simulink model "F18_sim_debug"  (R2025b)
settings: Solver=VariableStepAuto  StartTime=0.0  StopTime=10.0  RelTol=1e-3
undefined symbols (not defined in the file): F18
settings Model: Creator=deepa  LastModifiedBy=deepa

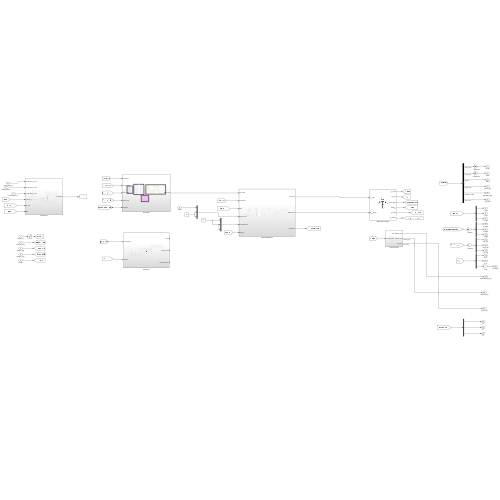
[thumbnail: Simulink's stored preview of the top-level diagram]
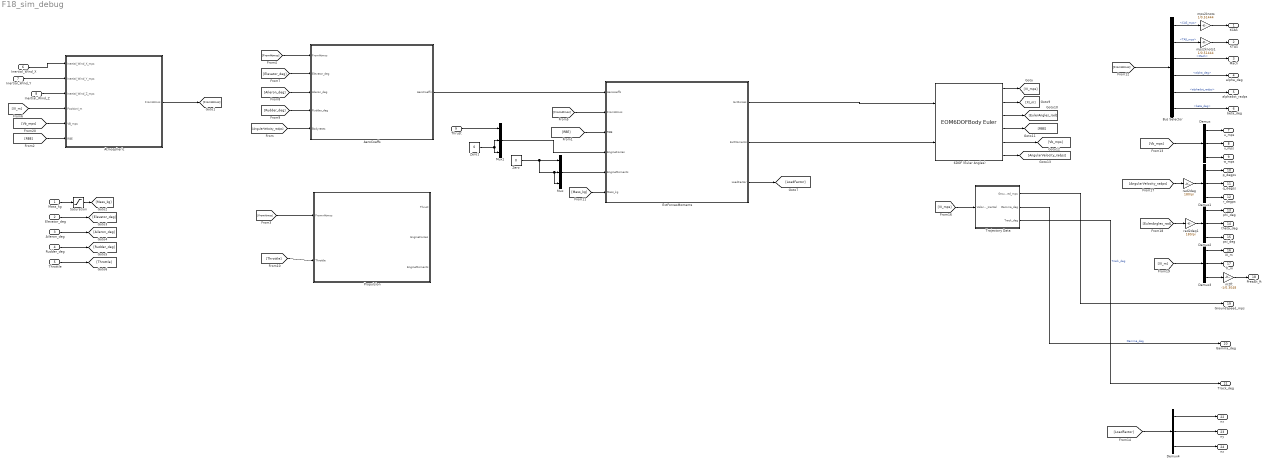
== system F18_sim_debug ==
  Mass_kg : Inport
  Elevator_deg : Inport  Port=2
  Aileron_deg : Inport  Port=3
  Rudder_deg : Inport  Port=4
  Throttle : Inport  Port=5
  Inertial_Wind_X : Inport  Port=6
  Inertial_Wind_Y : Inport  Port=7
  Inertial_Wind_Z : Inport  Port=8
  Thrust : Inport  Port=9
  6DOF (Euler Angles) : EOM6DOFBodyEuler  mass_0=15118.35  inertia=F18.Inertia  Vm_statename={'u_mps','v_mps','z_mps'}  xme_statename={'XI_m','YI_m','ZI_m'}  pm_statename={'p_radps','q_rapds','r_radps'}  eul_statename={'phi_rad','theta_rad','psi_rad'}
  AeroCoeffs : Subsystem
  Atmospheric : Subsystem
  Bus Selector : BusSelector  OutputSignals=CAS_mps,TAS_mps,Mach,alpha_deg,alphadot_radps,beta_deg
  Demux{,1..4} (5 alike) : Demux  Outputs=3
  ExtForcesMoments : Subsystem
  Mux : Mux  Inputs=3
  Mux1 : Mux  Inputs=3
  Propulsion : Subsystem
  Saturation : Saturate  UpperLimit=inf  LowerLimit=0.1
  Trajectory Data : Subsystem
  Zero : Constant  Value=0  OutDataTypeStr=Inherit: Inherit via back propagation
  Zero1 : Constant  Value=0  OutDataTypeStr=Inherit: Inherit via back propagation
  m2ft : Gain  Gain=-1/0.3048
  mps2knots : Gain  Gain=1/0.51444
  mps2knots1 : Gain  Gain=1/0.51444
  rad2deg : Gain  Gain=180/pi
  rad2deg1 : Gain  Gain=180/pi
  KCAS : Outport
  KTAS : Outport  Port=2
  Mach : Outport  Port=3
  alpha_deg : Outport  Port=4
  alphadot_radps : Outport  Port=5
  beta_deg : Outport  Port=6
  u_mps : Outport  Port=7
  v_mps : Outport  Port=8
  w_mps : Outport  Port=9
  p_degps : Outport  Port=10
  q_degps : Outport  Port=11
  r_degps : Outport  Port=12
  phi_deg : Outport  Port=13
  theta_deg : Outport  Port=14
  psi_deg : Outport  Port=15
  XI_m : Outport  Port=16
  YI_m : Outport  Port=17
  PresAlt_ft : Outport  Port=18
  GroundSpeed_mps : Outport  Port=19
  Gamma_deg : Outport  Port=20
  Track_deg : Outport  Port=21
  nx : Outport  Port=22
  ny : Outport  Port=23
  nz : Outport  Port=24
  wires:
  Bus Selector/3 -> Mach/1  "<Mach>"
  Saturation/1 -> [Mass_kg]
  Throttle/1 -> [Throttle]
  Aileron_deg/1 -> [Aileron_deg]
  [Elevator_deg] -> AeroCoeffs/2(Elevator_deg)
  Mass_kg/1 -> Saturation/1
  Inertial_Wind_X/1 -> Atmospheric/1(Inertial_Wind_X_mps)
  Trajectory Data/1(GroundSpeed_mps) -> GroundSpeed_mps/1
  [XI_m] -> Demux3/1
  AeroCoeffs/1(AeroCoeffs) -> ExtForcesMoments/1(Aerocoeffs)
  ExtForcesMoments/2(ExtMoments) -> 6DOF (Euler Angles)/2
  Demux2/3 -> psi_deg/1
  [Aileron_deg] -> AeroCoeffs/3(Aileron_deg)
  Bus Selector/1 -> mps2knots/1  "<CAS_mps>"
  Atmospheric/1(FromAtmos) -> [FromAtmos]
  Demux4/1 -> nx/1
  Demux1/3 -> r_degps/1
  rad2deg1/1 -> Demux2/1
  [LoadFactor] -> Demux4/1
  Rudder_deg/1 -> [Rudder_deg]
  Elevator_deg/1 -> [Elevator_deg]
  Demux3/1 -> XI_m/1
  Bus Selector/6 -> beta_deg/1  "<beta_deg>"
  Demux4/2 -> ny/1
  Demux3/2 -> YI_m/1
  Demux2/1 -> phi_deg/1
  Inertial_Wind_Y/1 -> Atmospheric/2(Inertial_Wind_Y_mps)
  Demux4/3 -> nz/1
  Bus Selector/4 -> alpha_deg/1  "<alpha_deg>"
  Demux3/3 -> m2ft/1
  Demux1/2 -> q_degps/1
  mps2knots/1 -> KCAS/1
  Inertial_Wind_Z/1 -> Atmospheric/3(Inertial_Wind_Z_mps)
  rad2deg/1 -> Demux1/1
  [Vb_mps] -> Demux/1
  [FromAtmos] -> Propulsion/1(FromnAtmos)
  Bus Selector/5 -> alphadot_radps/1  "<alphadot_radps>"
  [AngularVelocity_radps] -> rad2deg/1
  [EulerAngles_rad] -> rad2deg1/1
  [Mass_kg] -> ExtForcesMoments/6(Mass_kg)
  [Rudder_deg] -> AeroCoeffs/4(Rudder_deg)
  Demux/2 -> v_mps/1
  [RBE] -> ExtForcesMoments/3(RBE)
  [Throttle] -> Propulsion/2(Throttle)
  [FromAtmos] -> ExtForcesMoments/2(FromAtmos)
  [AngularVelocity_radps] -> AeroCoeffs/5(Bodyrates)
  Demux/3 -> w_mps/1
  ExtForcesMoments/3(LoadFactor) -> [LoadFactor]
  [FromAtmos] -> AeroCoeffs/1(FromAtmos)
  Demux1/1 -> p_degps/1
  Bus Selector/2 -> mps2knots1/1  "<TAS_mps>"
  m2ft/1 -> PresAlt_ft/1
  Demux/1 -> u_mps/1
  [FromAtmos] -> Bus Selector/1
  ExtForcesMoments/1(ExtForces) -> 6DOF (Euler Angles)/1
  Demux2/2 -> theta_deg/1
  mps2knots1/1 -> KTAS/1
  6DOF (Euler Angles)/1 -> [VI_mps]
  6DOF (Euler Angles)/2 -> [XI_m]
  6DOF (Euler Angles)/3 -> [EulerAngles_rad]
  6DOF (Euler Angles)/4 -> [RBE]
  6DOF (Euler Angles)/5 -> [Vb_mps]
  6DOF (Euler Angles)/6 -> [AngularVelocity_radps]
  [RBE] -> Atmospheric/6(RBE)
  [XI_m] -> Atmospheric/4(PositionI_m)
  [VI_mps] -> Trajectory Data/1(Velocity_Inertial)
  Trajectory Data/2(Gamma_deg) -> Gamma_deg/1  "Gamma_deg"
  Trajectory Data/3(Track_deg) -> Track_deg/1  "Track_deg"
  [Vb_mps] -> Atmospheric/5(VB_mps)
  Zero/1 -> Mux/3, Mux/2, Mux/1
  Mux/1 -> ExtForcesMoments/5(EngineMoments)
  Thrust/1 -> Mux1/1
  Zero1/1 -> Mux1/2, Mux1/3
  Mux1/1 -> ExtForcesMoments/4(EngineForces)

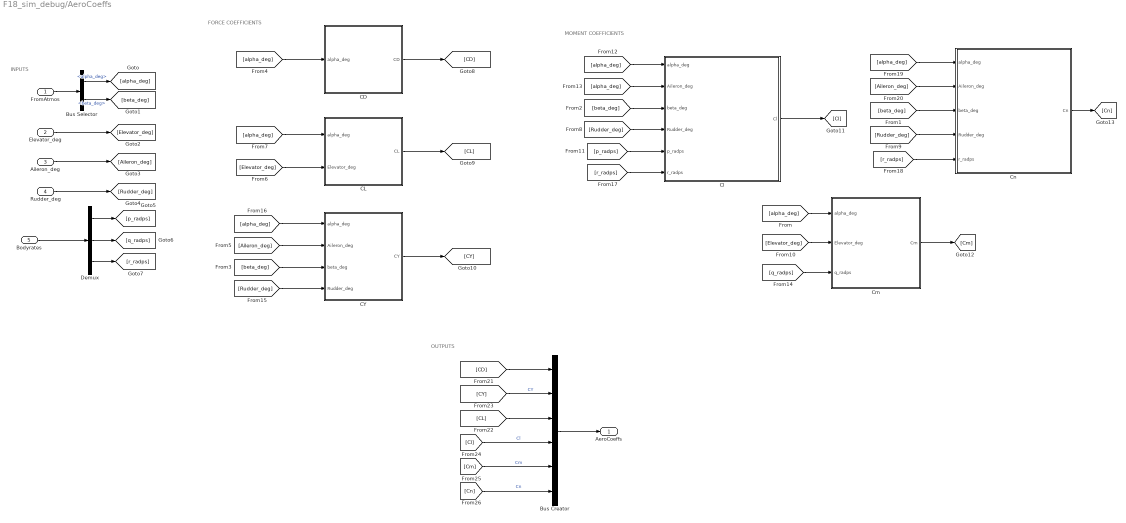
== system F18_sim_debug/AeroCoeffs ==
  note: OUTPUTS
  note: MOMENT COEFFICIENTS
  note: FORCE COEFFICIENTS
  note: INPUTS
  FromAtmos : Inport
  Elevator_deg : Inport  Port=2
  Aileron_deg : Inport  Port=3
  Rudder_deg : Inport  Port=4
  Bodyrates : Inport  Port=5
  Bus Creator : BusCreator  Inputs=6
  Bus Selector : BusSelector  OutputSignals=alpha_deg,beta_deg
  CD : Subsystem
  CL : Subsystem
  CY : Subsystem
  Cl : Subsystem
  Cm : Subsystem
  Cn : Subsystem
  Demux : Demux  Outputs=3
  AeroCoeffs : Outport
  wires:
  FromAtmos/1 -> Bus Selector/1
  [alpha_deg] -> Cm/1(alpha_deg)
  [beta_deg] -> Cn/3(beta_deg)
  [beta_deg] -> Cl/3(beta_deg)
  [beta_deg] -> CY/3(beta_deg)
  [alpha_deg] -> CD/1(alpha_deg)
  Elevator_deg/1 -> [Elevator_deg]
  Aileron_deg/1 -> [Aileron_deg]
  Rudder_deg/1 -> [Rudder_deg]
  [Aileron_deg] -> CY/2(Aileron_deg)
  [Elevator_deg] -> CL/2(Elevator_deg)
  [alpha_deg] -> CL/1(alpha_deg)
  [Rudder_deg] -> Cl/4(Rudder_deg)
  [Rudder_deg] -> Cn/4(Rudder_deg)
  [Elevator_deg] -> Cm/2(Elevator_deg)
  Bodyrates/1 -> Demux/1
  Demux/1 -> [p_radps]
  Demux/2 -> [q_radps]
  Demux/3 -> [r_radps]
  [p_radps] -> Cl/5(p_radps)
  [alpha_deg] -> Cl/1(alpha_deg)
  [alpha_deg] -> Cl/2(Aileron_deg)
  [q_radps] -> Cm/3(q_radps)
  [Rudder_deg] -> CY/4(Rudder_deg)
  [alpha_deg] -> CY/1(alpha_deg)
  [r_radps] -> Cl/6(r_radps)
  [r_radps] -> Cn/5(r_radps)
  [alpha_deg] -> Cn/1(alpha_deg)
  [Aileron_deg] -> Cn/2(Aileron_deg)
  CD/1(CD) -> [CD]
  CL/1(CL) -> [CL]
  CY/1(CY) -> [CY]
  Cl/1(Cl) -> [Cl]
  Cm/1(Cm) -> [Cm]
  Cn/1(Cn) -> [Cn]
  [CD] -> Bus Creator/1
  [CY] -> Bus Creator/2  "CY"
  [CL] -> Bus Creator/3
  [Cn] -> Bus Creator/6  "Cn"
  [Cm] -> Bus Creator/5  "Cm"
  [Cl] -> Bus Creator/4  "Cl"
  Bus Creator/1 -> AeroCoeffs/1
  Bus Selector/1 -> [alpha_deg]  "<alpha_deg>"
  Bus Selector/2 -> [beta_deg]  "<beta_deg>"

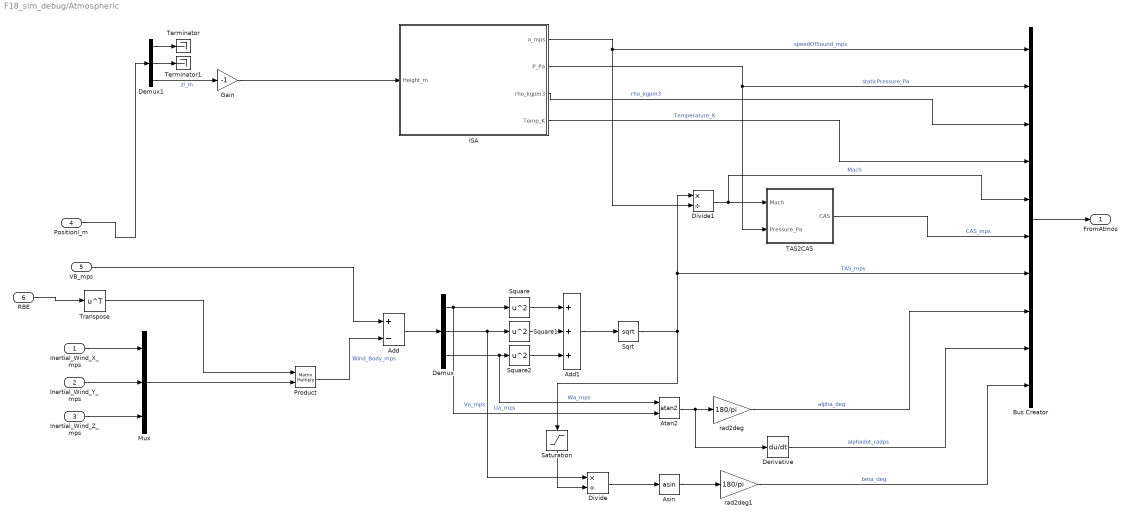
== system F18_sim_debug/Atmospheric ==
  Inertial_Wind_X_mps : Inport
  Inertial_Wind_Y_mps : Inport  Port=2
  Inertial_Wind_Z_mps : Inport  Port=3
  PositionI_m : Inport  Port=4
  VB_mps : Inport  Port=5
  RBE : Inport  Port=6
  Add : Sum  Inputs=+-
  Add1 : Sum  Inputs=+++
  Asin : Trigonometry  Operator=asin
  Atan2 : Trigonometry  Operator=atan2
  Bus Creator : BusCreator  Inputs=10
  Demux : Demux  Outputs=3
  Demux1 : Demux  Outputs=3
  Derivative : Derivative
  Divide : Product  Inputs=*/
  Divide1 : Product  Inputs=*/
  Gain : Gain  Gain=-1
  ISA : Subsystem
  Mux : Mux  Inputs=3
  Product : Product  Multiplication=Matrix(*)
  Saturation : Saturate  UpperLimit=inf  LowerLimit=0.1
  Sqrt : Sqrt
  Square : Math  Operator=square
  Square1 : Math  Operator=square
  Square2 : Math  Operator=square
  TAS2CAS : Subsystem
  Terminator : Terminator
  Terminator1 : Terminator
  Transpose : Math  Operator=transpose
  rad2deg : Gain  Gain=180/pi
  rad2deg1 : Gain  Gain=180/pi
  FromAtmos : Outport
  wires:
  Gain/1 -> ISA/1(Height_m)
  VB_mps/1 -> Add/1
  PositionI_m/1 -> Demux1/1
  Demux1/1 -> Terminator/1
  Demux1/2 -> Terminator1/1
  Demux1/3 -> Gain/1  "zI_m"
  Inertial_Wind_X_mps/1 -> Mux/1
  Inertial_Wind_Y_mps/1 -> Mux/2
  Inertial_Wind_Z_mps/1 -> Mux/3
  Transpose/1 -> Product/1
  Mux/1 -> Product/2
  Product/1 -> Add/2  "Wind_Body_mps"
  Add/1 -> Demux/1
  Demux/1 -> Square/1, Atan2/2  "Ua_mps"
  Demux/2 -> Square1/1, Divide/1  "Va_mps"
  Demux/3 -> Atan2/1, Square2/1  "Wa_mps"
  Square/1 -> Add1/1
  Square1/1 -> Add1/2
  Square2/1 -> Add1/3
  Add1/1 -> Sqrt/1
  Sqrt/1 -> Bus Creator/7, Divide1/1, Saturation/1  "TAS_mps"
  Atan2/1 -> Derivative/1, rad2deg/1
  rad2deg/1 -> Bus Creator/8  "alpha_deg"
  Divide/1 -> Asin/1
  Asin/1 -> rad2deg1/1
  rad2deg1/1 -> Bus Creator/10  "beta_deg"
  Derivative/1 -> Bus Creator/9  "alphadot_radps"
  ISA/1(a_mps) -> Divide1/2, Bus Creator/1  "speedOfSound_mps"
  Divide1/1 -> Bus Creator/5, TAS2CAS/1(Mach)  "Mach"
  ISA/2(P_Pa) -> TAS2CAS/2(Pressure_Pa), Bus Creator/2  "staticPressure_Pa"
  ISA/3(rho_kgpm3) -> Bus Creator/3  "rho_kgpm3"
  ISA/4(Temp_K) -> Bus Creator/4  "Temperature_K"
  TAS2CAS/1(CAS) -> Bus Creator/6  "CAS_mps"
  Bus Creator/1 -> FromAtmos/1
  Saturation/1 -> Divide/2
  RBE/1 -> Transpose/1

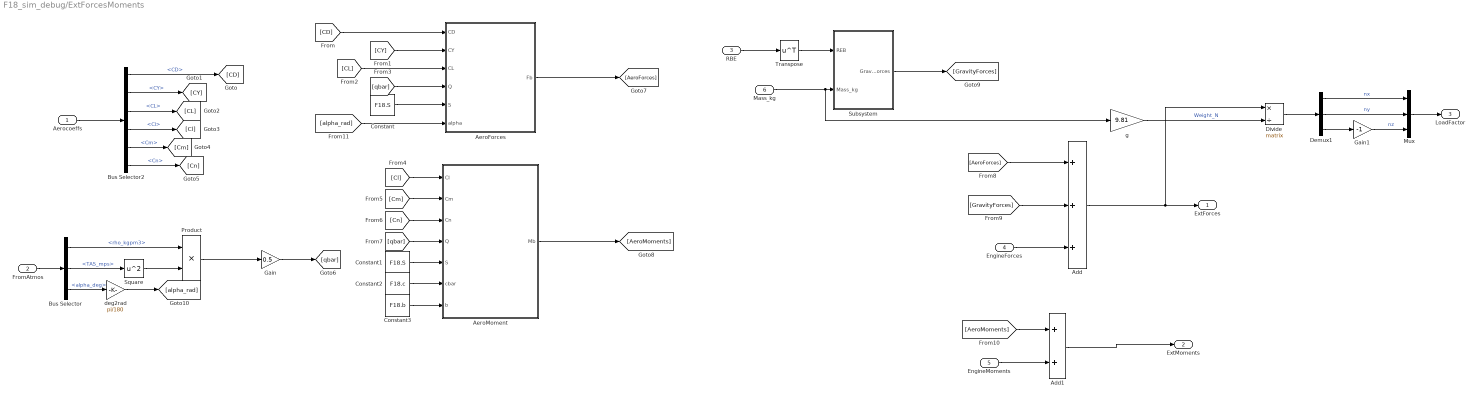
== system F18_sim_debug/ExtForcesMoments ==
  Aerocoeffs : Inport
  FromAtmos : Inport  Port=2
  RBE : Inport  Port=3
  EngineForces : Inport  Port=4
  EngineMoments : Inport  Port=5
  Mass_kg : Inport  Port=6
  Add : Sum  Inputs=+++
  Add1 : Sum
  AeroForces : MATLAB Function  TreatAsAtomicUnit=on
  AeroMoment : MATLAB Function  TreatAsAtomicUnit=on
  Bus Selector : BusSelector  OutputSignals=rho_kgpm3,TAS_mps,alpha_deg
  Bus Selector2 : BusSelector  OutputSignals=CD,CY,CL,Cl,Cm,Cn
  Constant : Constant  Value=F18.S
  Constant1 : Constant  Value=F18.S
  Constant2 : Constant  Value=F18.c
  Constant3 : Constant  Value=F18.b
  Demux1 : Demux  Outputs=3
  Divide : Product  Inputs=*/  Multiplication=Matrix(*)
  Gain : Gain  Gain=0.5
  Gain1 : Gain  Gain=-1
  Mux : Mux  Inputs=3
  Product : Product
  Square : Math  Operator=square
  Subsystem : Subsystem
  Transpose : Math  Operator=transpose
  deg2rad : Gain  Gain=pi/180
  g : Gain  Gain=9.81
  ExtForces : Outport
  ExtMoments : Outport  Port=2
  LoadFactor : Outport  Port=3
  wires:
  FromAtmos/1 -> Bus Selector/1
  Square/1 -> Product/2
  Product/1 -> Gain/1
  Gain/1 -> [qbar]
  [CY] -> AeroForces/2(CY)
  [CL] -> AeroForces/3(CL)
  Constant/1 -> AeroForces/5(S)
  [Cl] -> AeroMoment/1(Cl)
  [Cm] -> AeroMoment/2(Cm)
  [Cn] -> AeroMoment/3(Cn)
  [qbar] -> AeroMoment/4(Q)
  Constant1/1 -> AeroMoment/5(S)
  Constant2/1 -> AeroMoment/6(cbar)
  Constant3/1 -> AeroMoment/7(b)
  AeroForces/1(Fb) -> [AeroForces]
  AeroMoment/1(Mb) -> [AeroMoments]
  RBE/1 -> Transpose/1
  Transpose/1 -> Subsystem/1(REB)
  Subsystem/1(GravityForces) -> [GravityForces]
  [AeroForces] -> Add/1
  [GravityForces] -> Add/2
  EngineForces/1 -> Add/3
  [AeroMoments] -> Add1/1
  EngineMoments/1 -> Add1/2
  Add/1 -> Divide/1, ExtForces/1
  Add1/1 -> ExtMoments/1
  Bus Selector/1 -> Product/1  "<rho_kgpm3>"
  Bus Selector/2 -> Square/1  "<TAS_mps>"
  Mass_kg/1 -> g/1, Subsystem/2(Mass_kg)
  g/1 -> Divide/2  "Weight_N"
  Divide/1 -> Demux1/1
  Demux1/1 -> Mux/1  "nx"
  Demux1/2 -> Mux/2  "ny"
  Demux1/3 -> Gain1/1
  Gain1/1 -> Mux/3  "nz"
  Mux/1 -> LoadFactor/1
  [qbar] -> AeroForces/4(Q)
  [CD] -> AeroForces/1(CD)
  Aerocoeffs/1 -> Bus Selector2/1
  Bus Selector2/1 -> [CD]  "<CD>"
  Bus Selector2/2 -> [CY]  "<CY>"
  Bus Selector2/3 -> [CL]  "<CL>"
  Bus Selector2/4 -> [Cl]  "<Cl>"
  Bus Selector2/5 -> [Cm]  "<Cm>"
  Bus Selector2/6 -> [Cn]  "<Cn>"
  Bus Selector/3 -> deg2rad/1  "<alpha_deg>"
  deg2rad/1 -> [alpha_rad]
  [alpha_rad] -> AeroForces/6(alpha)

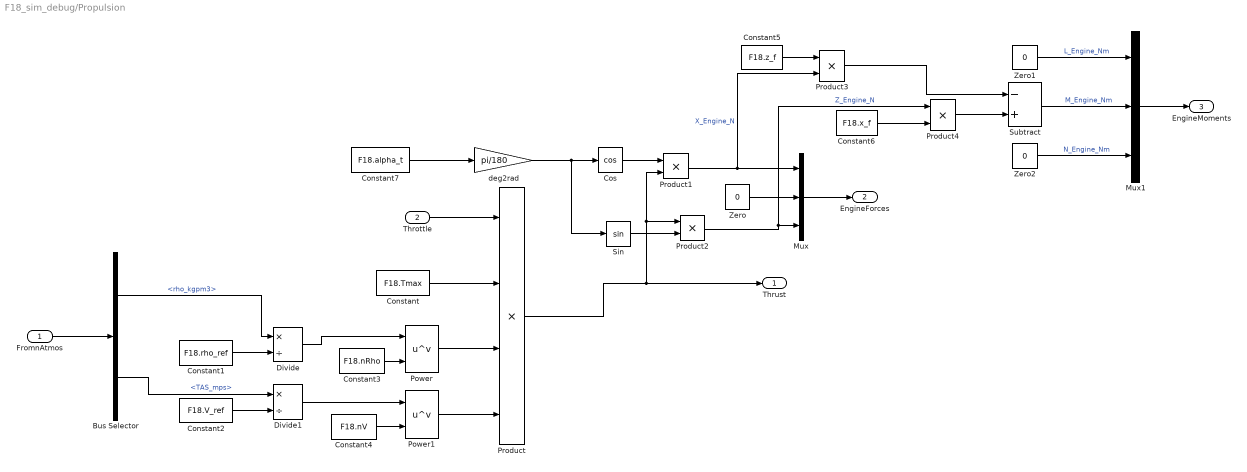
== system F18_sim_debug/Propulsion ==
  FromnAtmos : Inport
  Throttle : Inport  Port=2
  Bus Selector : BusSelector  OutputSignals=rho_kgpm3,TAS_mps
  Constant : Constant  Value=F18.Tmax
  Constant1 : Constant  Value=F18.rho_ref
  Constant2 : Constant  Value=F18.V_ref
  Constant3 : Constant  Value=F18.nRho
  Constant4 : Constant  Value=F18.nV
  Constant5 : Constant  Value=F18.z_f
  Constant6 : Constant  Value=F18.x_f
  Constant7 : Constant  Value=F18.alpha_t
  Cos : Trigonometry  Operator=cos
  Divide : Product  Inputs=*/
  Divide1 : Product  Inputs=*/
  Mux : Mux  Inputs=3
  Mux1 : Mux  Inputs=3
  Power : Math  Operator=pow
  Power1 : Math  Operator=pow
  Product : Product  Inputs=4
  Product{1..4} (4 alike) : Product
  Sin : Trigonometry
  Subtract : Sum  Inputs=-+
  Zero : Constant  Value=0  OutDataTypeStr=Inherit: Inherit via back propagation
  Zero1 : Constant  Value=0  OutDataTypeStr=Inherit: Inherit via back propagation
  Zero2 : Constant  Value=0  OutDataTypeStr=Inherit: Inherit via back propagation
  deg2rad : Gain  Gain=pi/180
  Thrust : Outport
  EngineForces : Outport  Port=2
  "EngineMoments " : Outport  Port=3
  wires:
  FromnAtmos/1 -> Bus Selector/1
  Bus Selector/1 -> Divide/1  "<rho_kgpm3>"
  Constant1/1 -> Divide/2
  Bus Selector/2 -> Divide1/1  "<TAS_mps>"
  Constant2/1 -> Divide1/2
  Divide/1 -> Power/1
  Divide1/1 -> Power1/1
  Constant3/1 -> Power/2
  Constant4/1 -> Power1/2
  Throttle/1 -> Product/1
  Constant/1 -> Product/2
  Power/1 -> Product/3
  Power1/1 -> Product/4
  Product/1 -> Thrust/1, Product2/1, Product1/2
  deg2rad/1 -> Sin/1, Cos/1
  Cos/1 -> Product1/1
  Product1/1 -> Product3/2, Mux/1  "X_Engine_N"
  Sin/1 -> Product2/2
  Product2/1 -> Product4/1, Mux/3  "Z_Engine_N"
  Zero/1 -> Mux/2
  Mux/1 -> EngineForces/1
  Constant5/1 -> Product3/1
  Constant6/1 -> Product4/2
  Product4/1 -> Subtract/2
  Product3/1 -> Subtract/1
  Subtract/1 -> Mux1/2  "M_Engine_Nm"
  Zero1/1 -> Mux1/1  "L_Engine_Nm"
  Zero2/1 -> Mux1/3  "N_Engine_Nm"
  Mux1/1 -> "EngineMoments "/1
  Constant7/1 -> deg2rad/1

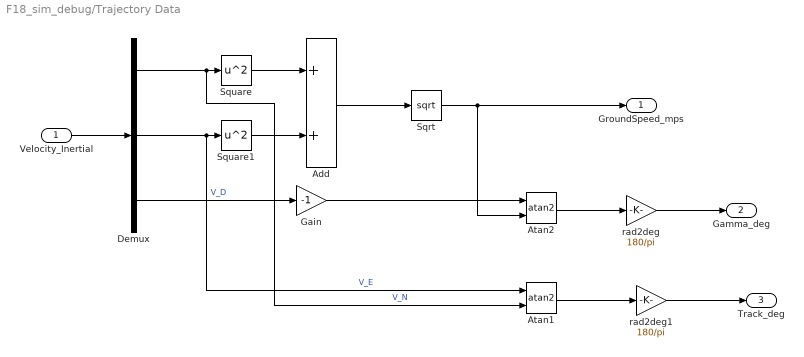
== system F18_sim_debug/Trajectory Data ==
  Velocity_Inertial : Inport
  Add : Sum
  Atan1 : Trigonometry  Operator=atan2
  Atan2 : Trigonometry  Operator=atan2
  Demux : Demux  Outputs=3
  Gain : Gain  Gain=-1
  Sqrt : Sqrt
  Square : Math  Operator=square
  Square1 : Math  Operator=square
  rad2deg : Gain  Gain=180/pi
  rad2deg1 : Gain  Gain=180/pi
  GroundSpeed_mps : Outport
  Gamma_deg : Outport  Port=2
  Track_deg : Outport  Port=3
  wires:
  rad2deg1/1 -> Track_deg/1
  Atan1/1 -> rad2deg1/1
  rad2deg/1 -> Gamma_deg/1
  Atan2/1 -> rad2deg/1
  Gain/1 -> Atan2/1
  Demux/3 -> Gain/1  "V_D"
  Sqrt/1 -> GroundSpeed_mps/1, Atan2/2
  Add/1 -> Sqrt/1
  Square1/1 -> Add/2
  Square/1 -> Add/1
  Demux/2 -> Square1/1, Atan1/1  "V_E"
  Demux/1 -> Square/1, Atan1/2  "V_N"
  Velocity_Inertial/1 -> Demux/1

== system F18_sim_debug/AeroCoeffs/CD ==
  alpha_deg : Inport
  MATLAB Function : MATLAB Function  TreatAsAtomicUnit=on
  Saturation : Saturate  UpperLimit=40  LowerLimit=-5
  CD : Outport
  wires:
  alpha_deg/1 -> Saturation/1
  MATLAB Function/1(CD) -> CD/1
  Saturation/1 -> MATLAB Function/1(alpha_deg)

== system F18_sim_debug/AeroCoeffs/CL ==
  alpha_deg : Inport
  Elevator_deg : Inport  Port=2
  MATLAB Function : MATLAB Function  TreatAsAtomicUnit=on
  Saturation : Saturate  UpperLimit=40  LowerLimit=-5
  Saturation1 : Saturate  UpperLimit=30  LowerLimit=-30
  CL : Outport
  wires:
  Saturation1/1 -> MATLAB Function/2(del_e_deg)
  Saturation/1 -> MATLAB Function/1(alpha_deg)
  Elevator_deg/1 -> Saturation1/1
  alpha_deg/1 -> Saturation/1
  MATLAB Function/1(CL) -> CL/1

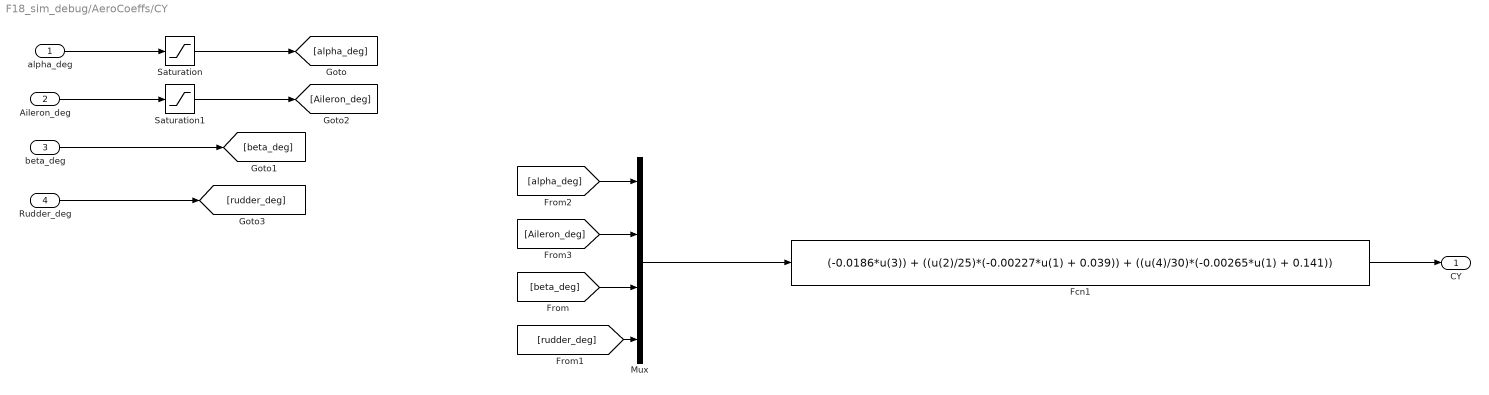
== system F18_sim_debug/AeroCoeffs/CY ==
  alpha_deg : Inport
  Aileron_deg : Inport  Port=2
  beta_deg : Inport  Port=3
  Rudder_deg : Inport  Port=4
  Fcn1 : Fcn  Expr=(-0.0186*u(3)) + ((u(2)/25)*(-0.00227*u(1) + 0.039)) + ((u(4)/30)*(-0.00265*u(1) + 0.141))
  Mux : Mux
  Saturation : Saturate  UpperLimit=35  LowerLimit=-5
  Saturation1 : Saturate  UpperLimit=40  LowerLimit=-5
  CY : Outport
  wires:
  [Aileron_deg] -> Mux/2
  [alpha_deg] -> Mux/1
  alpha_deg/1 -> Saturation/1
  Aileron_deg/1 -> Saturation1/1
  Fcn1/1 -> CY/1
  Saturation/1 -> [alpha_deg]
  Saturation1/1 -> [Aileron_deg]
  Mux/1 -> Fcn1/1
  beta_deg/1 -> [beta_deg]
  Rudder_deg/1 -> [rudder_deg]
  [beta_deg] -> Mux/3
  [rudder_deg] -> Mux/4

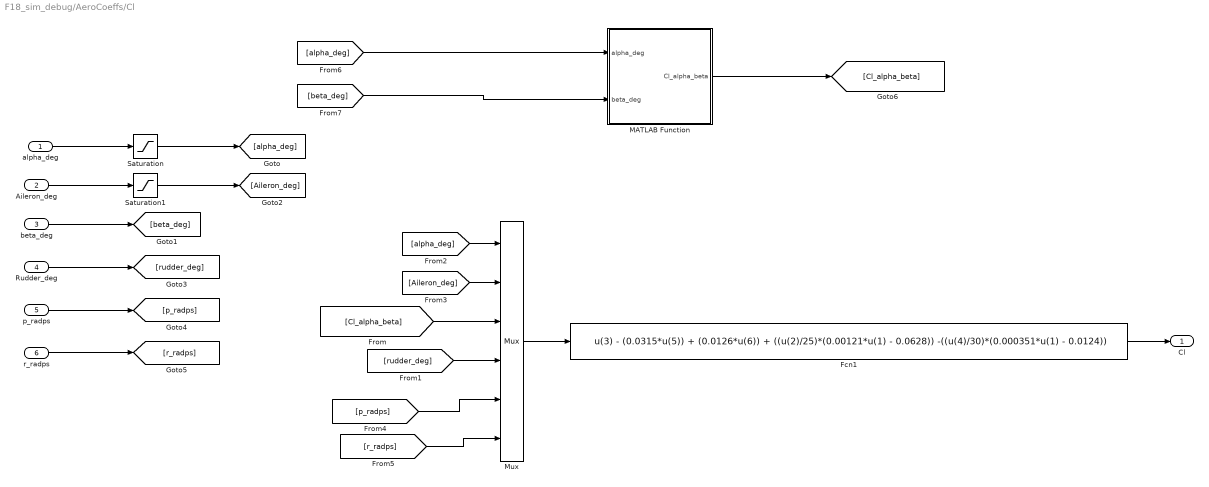
== system F18_sim_debug/AeroCoeffs/Cl ==
  alpha_deg : Inport
  Aileron_deg : Inport  Port=2
  beta_deg : Inport  Port=3
  Rudder_deg : Inport  Port=4
  p_radps : Inport  Port=5
  r_radps : Inport  Port=6
  Fcn1 : Fcn  Expr=u(3) - (0.0315*u(5)) + (0.0126*u(6)) + ((u(2)/25)*(0.00121*u(1) - 0.0628)) -((u(4)/30)*(0.000351*u(1) - 0.0124))
  MATLAB Function : MATLAB Function  TreatAsAtomicUnit=on
  Mux : Mux  Inputs=6
  Saturation : Saturate  UpperLimit=25  LowerLimit=-5
  Saturation1 : Saturate  UpperLimit=40  LowerLimit=-40
  Cl : Outport
  wires:
  [rudder_deg] -> Mux/4
  [Cl_alpha_beta] -> Mux/3
  Rudder_deg/1 -> [rudder_deg]
  beta_deg/1 -> [beta_deg]
  Mux/1 -> Fcn1/1
  Saturation1/1 -> [Aileron_deg]
  Saturation/1 -> [alpha_deg]
  Fcn1/1 -> Cl/1
  Aileron_deg/1 -> Saturation1/1
  alpha_deg/1 -> Saturation/1
  [alpha_deg] -> Mux/1
  [Aileron_deg] -> Mux/2
  p_radps/1 -> [p_radps]
  r_radps/1 -> [r_radps]
  [p_radps] -> Mux/5
  [r_radps] -> Mux/6
  [beta_deg] -> MATLAB Function/2(beta_deg)
  [alpha_deg] -> MATLAB Function/1(alpha_deg)
  MATLAB Function/1(Cl_alpha_beta) -> [Cl_alpha_beta]

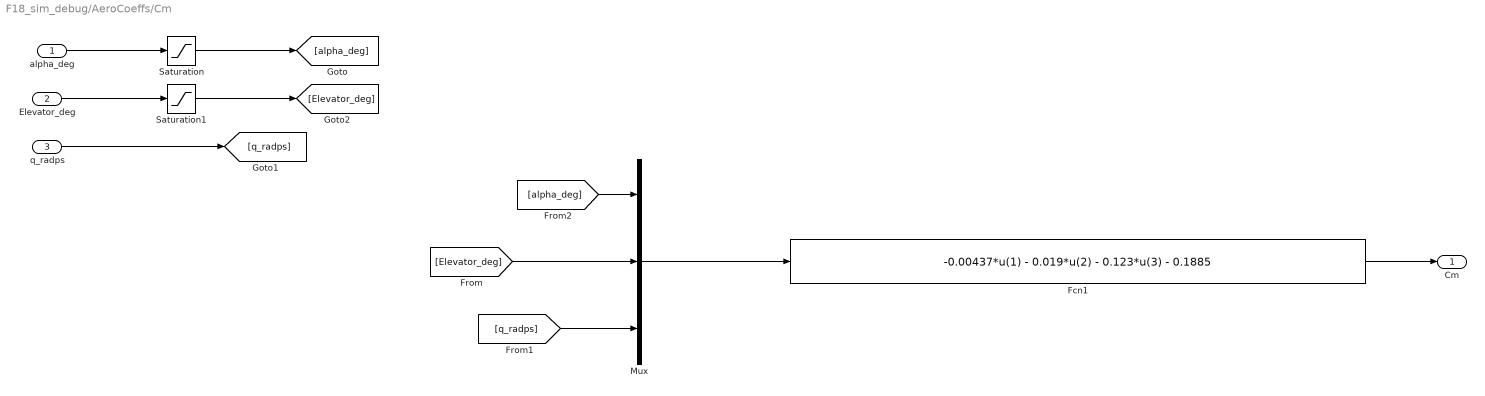
== system F18_sim_debug/AeroCoeffs/Cm ==
  alpha_deg : Inport
  Elevator_deg : Inport  Port=2
  q_radps : Inport  Port=3
  Fcn1 : Fcn  Expr=-0.00437*u(1) - 0.019*u(2) - 0.123*u(3) - 0.1885
  Mux : Mux  Inputs=3
  Saturation : Saturate  UpperLimit=40  LowerLimit=-5
  Saturation1 : Saturate  UpperLimit=40  LowerLimit=-5
  Cm : Outport
  wires:
  q_radps/1 -> [q_radps]
  Mux/1 -> Fcn1/1
  Saturation1/1 -> [Elevator_deg]
  Saturation/1 -> [alpha_deg]
  Fcn1/1 -> Cm/1
  Elevator_deg/1 -> Saturation1/1
  alpha_deg/1 -> Saturation/1
  [alpha_deg] -> Mux/1
  [Elevator_deg] -> Mux/2
  [q_radps] -> Mux/3

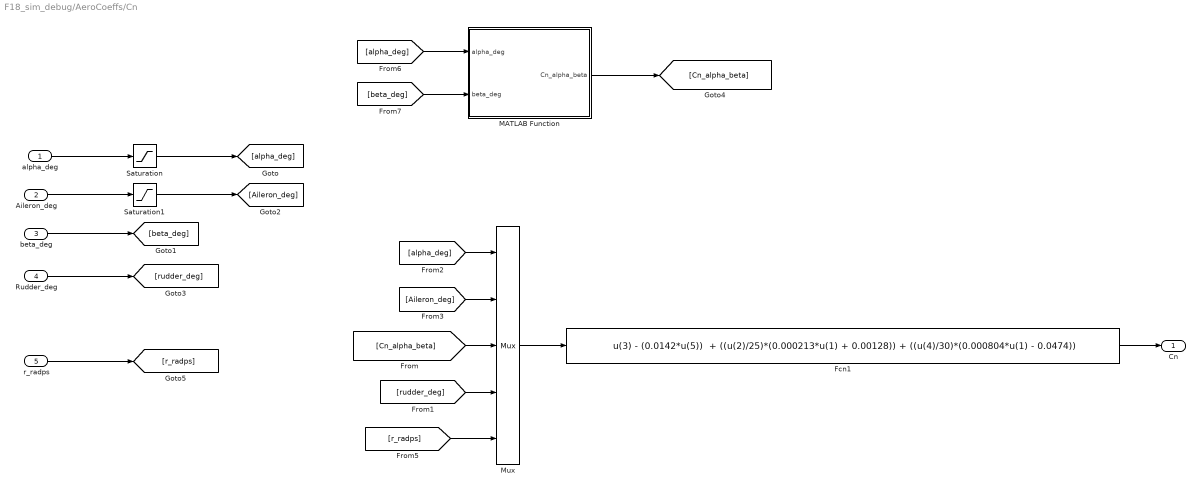
== system F18_sim_debug/AeroCoeffs/Cn ==
  alpha_deg : Inport
  Aileron_deg : Inport  Port=2
  beta_deg : Inport  Port=3
  Rudder_deg : Inport  Port=4
  r_radps : Inport  Port=5
  Fcn1 : Fcn  Expr="u(3) - (0.0142*u(5))  + ((u(2)/25)*(0.000213*u(1) + 0.00128)) + ((u(4)/30)*(0.000804*u(1) - 0.0474))"
  MATLAB Function : MATLAB Function  TreatAsAtomicUnit=on
  Mux : Mux  Inputs=5
  Saturation : Saturate  UpperLimit=35  LowerLimit=-5
  Saturation1 : Saturate  UpperLimit=40  LowerLimit=-5
  Cn : Outport
  wires:
  [beta_deg] -> MATLAB Function/2(beta_deg)
  [r_radps] -> Mux/5
  r_radps/1 -> [r_radps]
  [Aileron_deg] -> Mux/2
  [alpha_deg] -> Mux/1
  alpha_deg/1 -> Saturation/1
  Aileron_deg/1 -> Saturation1/1
  Fcn1/1 -> Cn/1
  Saturation/1 -> [alpha_deg]
  Saturation1/1 -> [Aileron_deg]
  Mux/1 -> Fcn1/1
  beta_deg/1 -> [beta_deg]
  Rudder_deg/1 -> [rudder_deg]
  [Cn_alpha_beta] -> Mux/3
  [rudder_deg] -> Mux/4
  [alpha_deg] -> MATLAB Function/1(alpha_deg)
  MATLAB Function/1(Cn_alpha_beta) -> [Cn_alpha_beta]

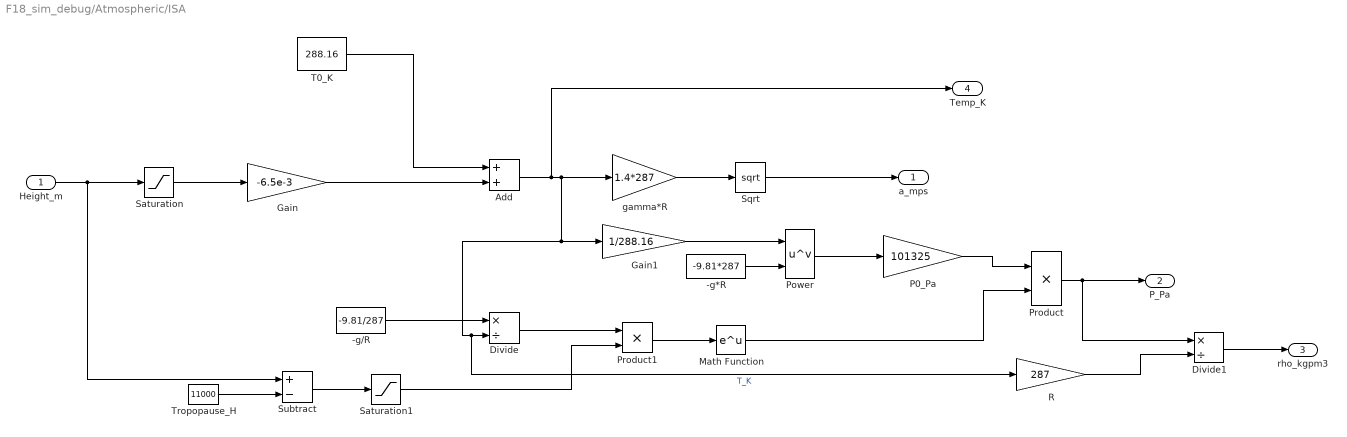
== system F18_sim_debug/Atmospheric/ISA ==
  Height_m : Inport
  " T0_K" : Constant  Value=288.16
  -g*R : Constant  Value=-9.81*287
  -g/R : Constant  Value=-9.81/287
  Add : Sum
  Divide : Product  Inputs=*/
  Divide1 : Product  Inputs=*/
  Gain : Gain  Gain=-6.5e-3
  Gain1 : Gain  Gain=1/288.16
  Math Function : Math
  P0_Pa : Gain  Gain=101325
  Power : Math  Operator=pow
  Product : Product
  Product1 : Product
  R : Gain  Gain=287
  Saturation : Saturate  UpperLimit=11000  LowerLimit=0
  Saturation1 : Saturate  UpperLimit=inf  LowerLimit=0
  Sqrt : Sqrt
  Subtract : Sum  Inputs=+-
  Tropopause_H : Constant  Value=11000
  gamma*R : Gain  Gain=1.4*287
  a_mps : Outport
  P_Pa : Outport  Port=2
  rho_kgpm3 : Outport  Port=3
  Temp_K : Outport  Port=4
  wires:
  Tropopause_H/1 -> Subtract/2
  gamma*R/1 -> Sqrt/1
  Sqrt/1 -> a_mps/1
  Add/1 -> Temp_K/1, gamma*R/1, R/1, Divide/2, Gain1/1  "T_K"
  Product1/1 -> Math Function/1
  Divide1/1 -> rho_kgpm3/1
  Product/1 -> P_Pa/1, Divide1/1
  Divide/1 -> Product1/1
  Math Function/1 -> Product/2
  Subtract/1 -> Saturation1/1
  Height_m/1 -> Subtract/1, Saturation/1
  Power/1 -> P0_Pa/1
  -g/R/1 -> Divide/1
  " T0_K"/1 -> Add/1
  Gain/1 -> Add/2
  R/1 -> Divide1/2
  P0_Pa/1 -> Product/1
  Saturation/1 -> Gain/1
  Saturation1/1 -> Product1/2
  -g*R/1 -> Power/2
  Gain1/1 -> Power/1

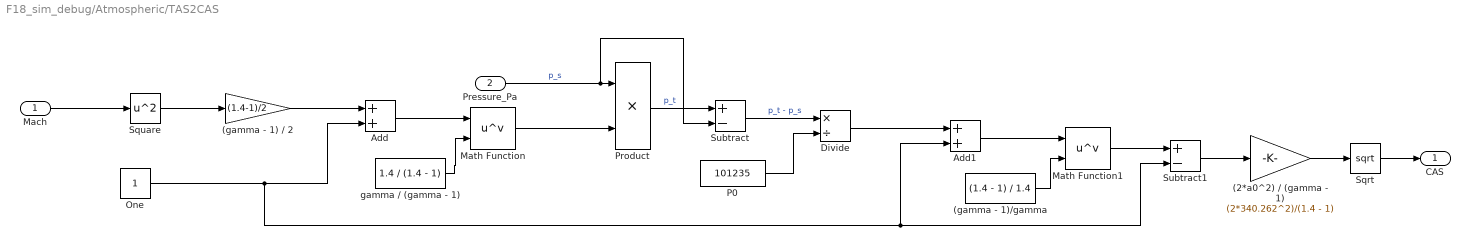
== system F18_sim_debug/Atmospheric/TAS2CAS ==
  Mach : Inport
  Pressure_Pa : Inport  Port=2
  (2*a0^2) / (gamma - 1) : Gain  Gain=(2*340.262^2)/(1.4 - 1)
  (gamma - 1) / 2 : Gain  Gain=(1.4-1)/2
  (gamma - 1)/gamma : Constant  Value=(1.4 - 1) / 1.4
  Add : Sum
  Add1 : Sum
  Divide : Product  Inputs=*/
  Math Function : Math  Operator=pow
  Math Function1 : Math  Operator=pow
  One : Constant  OutDataTypeStr=Inherit: Inherit via back propagation
  P0 : Constant  Value=101235
  Product : Product
  Sqrt : Sqrt
  Square : Math  Operator=square
  Subtract : Sum  Inputs=+-
  Subtract1 : Sum  Inputs=+-
  gamma / (gamma - 1) : Constant  Value=1.4 / (1.4 - 1)
  CAS : Outport
  wires:
  Mach/1 -> Square/1
  Square/1 -> (gamma - 1) / 2/1
  One/1 -> Subtract1/2, Add1/2, Add/2
  (gamma - 1) / 2/1 -> Add/1
  Add/1 -> Math Function/1
  gamma / (gamma - 1)/1 -> Math Function/2
  Pressure_Pa/1 -> Subtract/2, Product/1  "p_s"
  Math Function/1 -> Product/2
  Product/1 -> Subtract/1  "p_t"
  Subtract/1 -> Divide/1  "p_t - p_s"
  P0/1 -> Divide/2
  Divide/1 -> Add1/1
  Add1/1 -> Math Function1/1
  (gamma - 1)/gamma/1 -> Math Function1/2
  Math Function1/1 -> Subtract1/1
  Subtract1/1 -> (2*a0^2) / (gamma - 1)/1
  Sqrt/1 -> CAS/1
  (2*a0^2) / (gamma - 1)/1 -> Sqrt/1

== system F18_sim_debug/ExtForcesMoments/Subsystem ==
  REB : Inport
  Mass_kg : Inport  Port=2
  Constant : Constant  Value=0
  Constant1 : Constant  Value=0
  Mux : Mux  Inputs=3
  Product : Product  Multiplication=Matrix(*)
  g : Gain  Gain=9.81
  GravityForces : Outport
  wires:
  Constant/1 -> Mux/1
  Constant1/1 -> Mux/2
  g/1 -> Mux/3
  REB/1 -> Product/1
  Mux/1 -> Product/2
  Product/1 -> GravityForces/1
  Mass_kg/1 -> g/1

== matlab function F18_sim_debug/AeroCoeffs/Cn/MATLAB Function ==
  data: alpha_deg input; Cn_alpha_beta output; beta_deg input
function Cn_alpha_beta = fcn(alpha_deg, beta_deg)

Delta = deg2rad(2);   
alpha = deg2rad(alpha_deg);
w1 = 0.5*(1 + tanh((alpha - deg2rad(10))/Delta));
w2 = 0.5*(1 + tanh((alpha - deg2rad(25))/Delta));

% Regime models
f1 = 0.00125;
f2 = -0.00022*alpha + 0.00342;
f3 = -0.0020;

% Smooth combination
f_alpha = (1 - w1)*f1 + w1*(1 - w2)*f2 + w2*f3;

Cn_alpha_beta = beta_deg * f_alpha;
end

== matlab function F18_sim_debug/ExtForcesMoments/AeroForces ==
  data: CD input double; Fb output; CY input; CL input; Q input; S input; alpha input
function Fb = Forces(CD, CY, CL, Q, S, alpha)

    D = Q*S*CD;
    Y = Q*S*CY;
    L = Q*S*CL;

    Fs = [-D; Y; -L];

    %Rotate these forces to F_b (body axis)
    RSB = [cos(alpha) 0 -sin(alpha);
        0 1 0;
        sin(alpha) 0 cos(alpha)];

    Fb = RSB*Fs;
    
end

== matlab function F18_sim_debug/ExtForcesMoments/AeroMoment ==
  data: Cl input; Mb output; Cm input; Cn input; Q input; S input; cbar input; b input
function Mb = Moments(Cl, Cm, Cn, Q, S, cbar, b)

    L = Q*S*Cl*b;
    M = Q*S*Cm*cbar;
    N = Q*S*Cn*b;

   Mb = [L; M; N];

end

== matlab function F18_sim_debug/AeroCoeffs/CL/MATLAB Function ==
  data: alpha_deg input; CL output double; del_e_deg input
function  CL = fcn(alpha_deg, del_e_deg)

alpha = deg2rad(alpha_deg);
alpha0 = deg2rad(10);
delta = deg2rad(2);

w = 0.5*(1 + (tanh((alpha - alpha0)/delta)));

CL_low = 0.0752*alpha_deg + 0.0144*del_e_deg + 0.732;
CL_high = -0.00148*alpha_deg^2 - 0.106*alpha_deg + 0.0144*del_e_deg + 0.569;

CL = ((1-w)*CL_low) + (w*CL_high);

end

== matlab function F18_sim_debug/AeroCoeffs/CD/MATLAB Function ==
  data: alpha_deg input; CD output double
function CD = fcn(alpha_deg)

alpha = deg2rad(alpha_deg);
alpha0 = deg2rad(20);
delta = deg2rad(2);

w = 0.5*(1 + (tanh((alpha - alpha0)/delta)));

CD_low = -0.0000348*alpha_deg^2 + 0.0473*alpha_deg - 0.3358;
CD_high = 0.0013*alpha_deg^2 - 0.00438*alpha_deg + 0.1423;

CD = ((1-w)*CD_low) + (w*CD_high);

end

== matlab function F18_sim_debug/AeroCoeffs/Cl/MATLAB Function ==
  data: alpha_deg input; Cl_alpha_beta output; beta_deg input
function Cl_alpha_beta = fcn(alpha_deg, beta_deg)

alpha = deg2rad(alpha_deg);
alpha0 = deg2rad(15);
delta = deg2rad(2);

w = 0.5*(1 + (tanh((alpha - alpha0)/delta)));

Cl_alpha_beta_low = -0.00012*alpha_deg - 0.00092;
Cl_alpha_beta_high = 0.00022*alpha_deg - 0.006;

Cl_alpha_beta = beta_deg*((1-w)*Cl_alpha_beta_low + w*Cl_alpha_beta_high);

end
